simulink model "model_3_nadoby"  (Simulink 5.0)
settings: Solver=ode45  StartTime=0.0  StopTime=300  RelTol=1e-3
values from neighbouring files (symbols this model uses):
  A =     [bcc.mat]    (also in hydrostart.m = 0.001)
  q_max1 = max(Q1_arr)    [ident_pump1_all_data.m]    (also in pump1-2009-12--2-17-54-58.mat = 2.57369035514e-05; pump1-2009-12--2-19--4--9.mat = 1.7227084293e-05; pump1-2009-12--3--8-53-53.mat = 1.75961801886e-05; pump1-2010--1--7-18-33--0.mat = 1.76359538152e-05)
  q_max2 = 2.60914737436e-05    [pump2-2009-12--2-18--7--0.mat]    (also in pump2-2009-12--2-19-16-16.mat = 1.73913043478e-05; pump2-2009-12--3--9-22-13.mat = 1.7316017316e-05; pump2-2010--1-25-13-52-28.mat = 1.72192916353e-05; pump2-2010--1-25-20--0-32.mat = 4.61836580902e-06)
undefined symbols (not defined in the file or in its folder): b1, b12, b2, b23, b3, lev1_init, lev2_init, lev3_init, posun1, posun2, posun3, prepni, q1_percenta, q2_percenta, q3_percenta
settings Model: LastModifiedBy=student  SignalLoggingName=logsout  RTWOptions="-aEnforceIntegerDowncast=1 -aFoldNonRolledExpr=1 -aInlineInvariantSignals=1 -aInlineParameters=0 -aLocalBlockOutputs=1 -aRollThreshold=5 -aZeroInternalMemoryAtStartup=1 -aZeroExternalMemoryAtStartup=1 -aInitFltsAndDblsToZero=1 -aGenerateReport=0 -aGenCodeOnly=0 -aRTWVerbose=1 -aIncludeHyperlinkInReport=0 -aLaunchReport=0 -aForceParamTrailComments=0 -aGenerateComments=1 -aIgnoreCustomStorageClasses=1 -aIncHierarchyInIds=0 -aMaxRTWIdLen=31 -aShowEliminatedStatements=0 -aPrefixModelToSubsysFcnNames=1 -aIncDataTypeInIds=0 -aInsertBlockDesc=0 -aSimulinkBlockComments=1 -aInlinedPrmAccess=\"Literals\"  -aSuppressErrorStatus=0 -aModelReferenceCompliant=1 -aSupportNonInlinedSFcns=1 -aSupportContinuousTime=1 -aSupportComplex=1 -aSupportNonFinite=1 -aSupportAbsoluteTime=1 -aTargetFcnLib=\"ansi_tfl_tmw.mat\" -aMultiInstanceERTCode=0 -aLogVarNameModifier=\"rt_\" -aIsPILTarget=0 -aCombineOutputUpdateFcns=0 -aGenerateASAP2=0 -aGenerateSampleERTMain=0 -aGenerateFullHeader=1 -aUtilityFuncGeneration=\"Auto\" -aIncludeFileDelimiter=\"Auto\" -aIncludeMdlTerminateFcn=1 -aPurelyIntegerCode=0 -aERTCustomFileBanners=0 -aRTWCAPIStates=0 -aRTWCAPIParams=0 -aRTWCAPISignals=0 -aMatFileLogging=1 -aGenFloatMathFcnCalls=\"ANSI_C\" -aExtModeMexFile=\"ext_comm\" -aExtModeTransport=0 -aExtModeStaticAllocSize=1000000 -aExtModeTesting=0 -aExtModeStaticAlloc=0 -aExtMode=0"

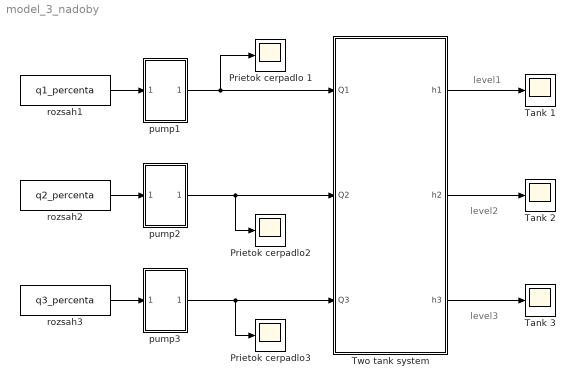
== system model_3_nadoby ==
  note: level1
  note: level2
  note: level3
  Prietok cerpadlo 1 : Scope
      settings: YMin=-5e-031  YMax=3.25e-030  SaveName=q1s  DataFormat=Array  SampleInput=on
  Prietok cerpadlo2 : Scope
      settings: YMin=-5e-031  YMax=3.25e-030  SaveName=q1s1  DataFormat=Array  SampleInput=on
  Prietok cerpadlo3 : Scope
      settings: YMin=-5e-031  YMax=3.25e-030  SaveName=q1s2  DataFormat=Array  SampleInput=on
  Tank 1 : Scope
      settings: YMin=-5e-031  YMax=3.25e-030  SaveName=h1s  DataFormat=Array  SampleInput=on
  Tank 2 : Scope
      settings: YMin=-5e-031  YMax=3.25e-030  SaveName=h2s  DataFormat=Array  SampleInput=on
  Tank 3 : Scope
      settings: YMin=-5e-031  YMax=3.25e-030  SaveName=h3s  DataFormat=Array  SampleInput=on
  Two tank system : Subsystem  TreatAsAtomicUnit=on
  pump1 : Subsystem
  pump2 : Subsystem
  pump3 : Subsystem
  rozsah1 : Constant  Value=q1_percenta
  rozsah2 : Constant  Value=q2_percenta
  rozsah3 : Constant  Value=q3_percenta
  wires:
  Two tank system/1(h1) -> Tank 1/1
  rozsah1/1 -> pump1/1(In1)
  pump1/1(Out1) -> Two tank system/1(Q1), Prietok cerpadlo 1/1
  rozsah2/1 -> pump2/1(In1)
  pump2/1(Out1) -> Prietok cerpadlo2/1, Two tank system/2(Q2)
  Two tank system/2(h2) -> Tank 2/1
  rozsah3/1 -> pump3/1(In1)
  pump3/1(Out1) -> Prietok cerpadlo3/1, Two tank system/3(Q3)
  Two tank system/3(h3) -> Tank 3/1

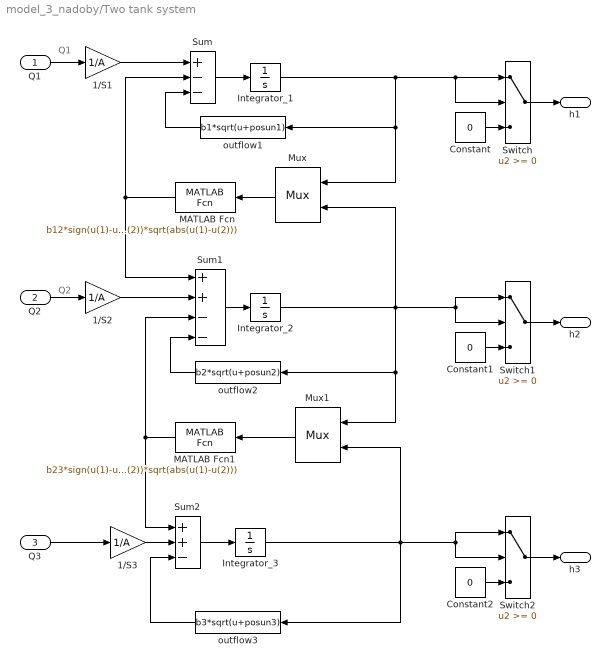
== system model_3_nadoby/Two tank system ==
  note: Q1
  note: Q2
  Q1 : Inport
  Q2 : Inport  Port=2
  Q3 : Inport  Port=3
  1/S1 : Gain  Gain=1/A  SaturateOnIntegerOverflow=on
  1/S2 : Gain  Gain=1/A  SaturateOnIntegerOverflow=on
  1/S3 : Gain  Gain=1/A  SaturateOnIntegerOverflow=on
  Constant : Constant  Value=0
  Constant1 : Constant  Value=0
  Constant2 : Constant  Value=0
  Integrator_1 : Integrator  InitialCondition=lev1_init  LimitOutput=on  UpperSaturationLimit=0.26  LowerSaturationLimit=0
  Integrator_2 : Integrator  InitialCondition=lev2_init  LimitOutput=on  UpperSaturationLimit=0.26  LowerSaturationLimit=0
  Integrator_3 : Integrator  InitialCondition=lev3_init  LimitOutput=on  UpperSaturationLimit=0.26  LowerSaturationLimit=0
  MATLAB Fcn : MATLABFcn  Orientation=left  MATLABFcn=b12*sign(u(1)-u(2))*sqrt(abs(u(1)-u(2)))  OutputSignalType=real
  MATLAB Fcn1 : MATLABFcn  Orientation=left  MATLABFcn=b23*sign(u(1)-u(2))*sqrt(abs(u(1)-u(2)))  OutputSignalType=real
  Mux : Mux  Orientation=left  Inputs=2
      settings: DisplayOption=signals
  Mux1 : Mux  Orientation=left  Inputs=2
      settings: DisplayOption=signals
  Sum : Sum  Inputs=+--  SaturateOnIntegerOverflow=on  InputSameDT=on
  Sum1 : Sum  Inputs=++--  SaturateOnIntegerOverflow=on  InputSameDT=on
  Sum2 : Sum  Inputs=++-  SaturateOnIntegerOverflow=on  InputSameDT=on
  Switch : Switch  SaturateOnIntegerOverflow=on
  Switch1 : Switch  SaturateOnIntegerOverflow=on
  Switch2 : Switch  SaturateOnIntegerOverflow=on
  outflow1 : Fcn  Orientation=left  Expr=b1*sqrt(u+posun1)
  outflow2 : Fcn  Orientation=left  Expr=b2*sqrt(u+posun2)
  outflow3 : Fcn  Orientation=left  Expr=b3*sqrt(u+posun3)
  h1 : Outport
  h2 : Outport  Port=2
  h3 : Outport  Port=3
  wires:
  1/S1/1 -> Sum/1
  Sum/1 -> Integrator_1/1
  Constant/1 -> Switch/3
  Switch/1 -> h1/1
  Q1/1 -> 1/S1/1
  Integrator_1/1 -> Switch/1, Switch/2, outflow1/1, Mux/1
  Q2/1 -> 1/S2/1
  Constant1/1 -> Switch1/3
  Switch1/1 -> h2/1
  Integrator_2/1 -> Switch1/2, Switch1/1, Mux/2, outflow2/1, Mux1/1
  outflow1/1 -> Sum/3
  Sum1/1 -> Integrator_2/1
  1/S2/1 -> Sum1/2
  MATLAB Fcn/1 -> Sum/2, Sum1/1
  Mux/1 -> MATLAB Fcn/1
  Q3/1 -> 1/S3/1
  outflow2/1 -> Sum1/4
  1/S3/1 -> Sum2/2
  Sum2/1 -> Integrator_3/1
  Integrator_3/1 -> outflow3/1, Mux1/2, Switch2/1, Switch2/2
  outflow3/1 -> Sum2/3
  Mux1/1 -> MATLAB Fcn1/1
  MATLAB Fcn1/1 -> Sum1/3, Sum2/1
  Constant2/1 -> Switch2/3
  Switch2/1 -> h3/1

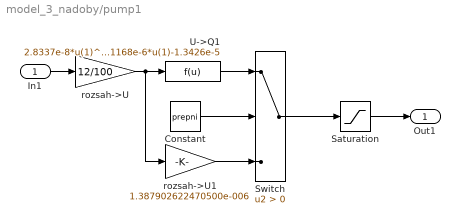
== system model_3_nadoby/pump1 ==
  In1 : Inport
  Constant : Constant  Value=prepni
  Saturation : Saturate  UpperLimit=q_max1  LowerLimit=0
  Switch : Switch  Criteria=u2 > Threshold  SaturateOnIntegerOverflow=on
  U->Q1 : Fcn  Expr=2.8337e-8*u(1)^3-8.0615e-7*u(1)^2+8.1168e-6*u(1)-1.3426e-5
  rozsah->U : Gain  Gain=12/100  SaturateOnIntegerOverflow=on
  rozsah->U1 : Gain  Gain=1.387902622470500e-006  SaturateOnIntegerOverflow=on
  Out1 : Outport
  wires:
  rozsah->U/1 -> U->Q1/1, rozsah->U1/1
  Constant/1 -> Switch/2
  U->Q1/1 -> Switch/1
  rozsah->U1/1 -> Switch/3
  In1/1 -> rozsah->U/1
  Switch/1 -> Saturation/1
  Saturation/1 -> Out1/1

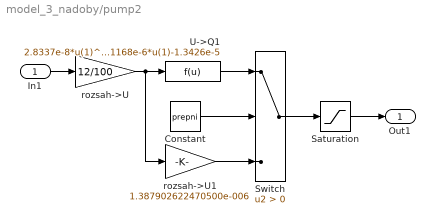
== system model_3_nadoby/pump2 ==
  In1 : Inport
  Constant : Constant  Value=prepni
  Saturation : Saturate  UpperLimit=q_max2  LowerLimit=0
  Switch : Switch  Criteria=u2 > Threshold  SaturateOnIntegerOverflow=on
  U->Q1 : Fcn  Expr=2.8337e-8*u(1)^3-8.0615e-7*u(1)^2+8.1168e-6*u(1)-1.3426e-5
  rozsah->U : Gain  Gain=12/100  SaturateOnIntegerOverflow=on
  rozsah->U1 : Gain  Gain=1.387902622470500e-006  SaturateOnIntegerOverflow=on
  Out1 : Outport
  wires:
  In1/1 -> rozsah->U/1
  rozsah->U1/1 -> Switch/3
  U->Q1/1 -> Switch/1
  Constant/1 -> Switch/2
  rozsah->U/1 -> rozsah->U1/1, U->Q1/1
  Switch/1 -> Saturation/1
  Saturation/1 -> Out1/1

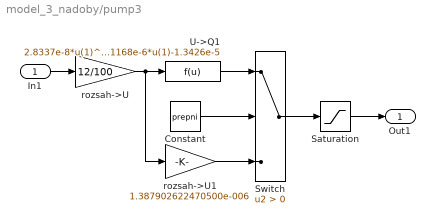
== system model_3_nadoby/pump3 ==
  In1 : Inport
  Constant : Constant  Value=prepni
  Saturation : Saturate  UpperLimit=q_max2  LowerLimit=0
  Switch : Switch  Criteria=u2 > Threshold  SaturateOnIntegerOverflow=on
  U->Q1 : Fcn  Expr=2.8337e-8*u(1)^3-8.0615e-7*u(1)^2+8.1168e-6*u(1)-1.3426e-5
  rozsah->U : Gain  Gain=12/100  SaturateOnIntegerOverflow=on
  rozsah->U1 : Gain  Gain=1.387902622470500e-006  SaturateOnIntegerOverflow=on
  Out1 : Outport
  wires:
  Saturation/1 -> Out1/1
  Switch/1 -> Saturation/1
  rozsah->U/1 -> U->Q1/1, rozsah->U1/1
  Constant/1 -> Switch/2
  U->Q1/1 -> Switch/1
  rozsah->U1/1 -> Switch/3
  In1/1 -> rozsah->U/1
